simulink library "EOM_lib"  (R2015a)
settings: Solver=ode45  StartTime=0.0  StopTime=10.0  RelTol=1e-3
undefined symbols (not defined in the file): EOM
libraries: aerolibutil x4, aerolib6dof2 x1
settings Model: Creator=Andrew  LastModifiedBy=Andrew

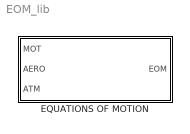
== system EOM_lib ==
  EQUATIONS OF MOTION : Subsystem

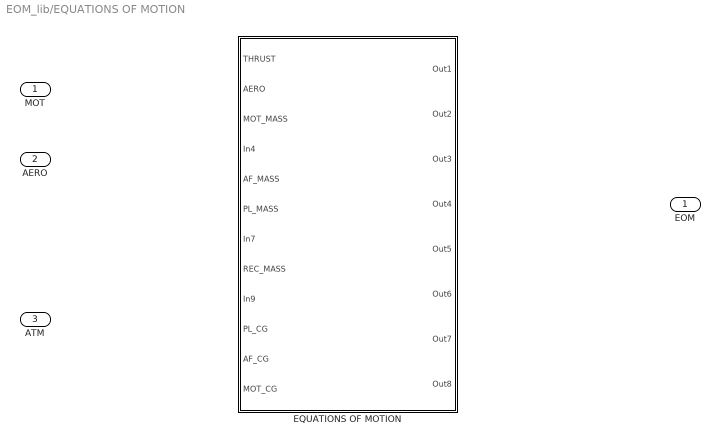
== system EOM_lib/EQUATIONS OF MOTION ==
  MOT : Inport
  AERO : Inport  Port=2
  ATM : Inport  Port=3
  EQUATIONS OF MOTION : Subsystem
  EOM : Outport

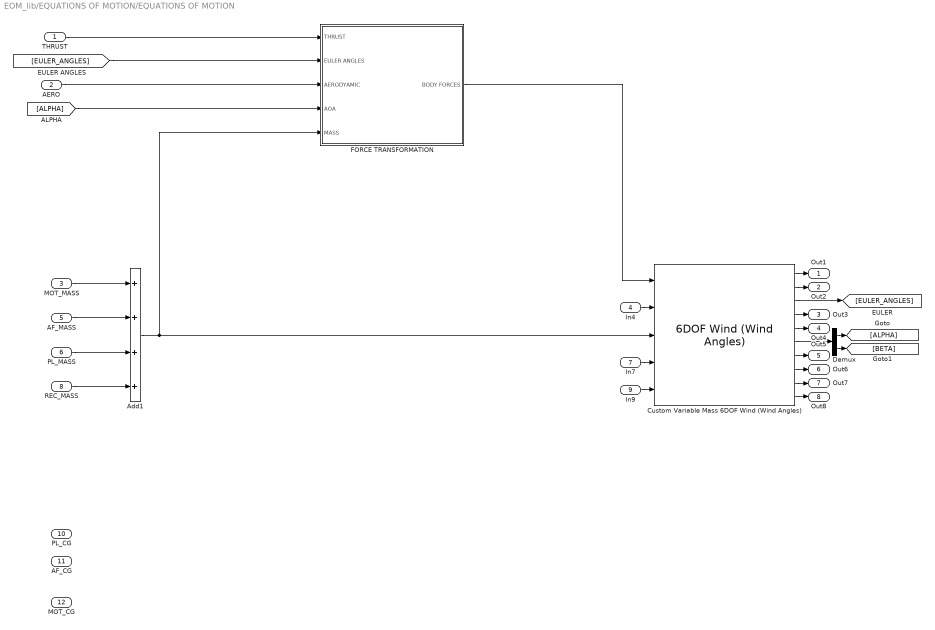
== system EOM_lib/EQUATIONS OF MOTION/EQUATIONS OF MOTION ==
  THRUST : Inport
  AERO : Inport  Port=2
  MOT_MASS : Inport  Port=3
  In4 : Inport  Port=4
  AF_MASS : Inport  Port=5
  PL_MASS : Inport  Port=6
  In7 : Inport  Port=7
  REC_MASS : Inport  Port=8
  In9 : Inport  Port=9
  PL_CG : Inport  Port=10
  AF_CG : Inport  Port=11
  MOT_CG : Inport  Port=12
  Add1 : Sum  Inputs=++++
  Custom Variable Mass 6DOF Wind (Wind Angles) : aerolib6dof2/6DOF Wind (Wind Angles)  units=Metric (MKS)  mtype=Custom Variable  rep=Wind Angles  xme_0=[0 0 0]  Vm_0=[0 0 0]  wind_0=[0 0 0]  pm_0=[0 0 0]  mass_0=1.0  mass_e=0.5  mass_f=2.0  inertia=eye(3)  inertia_e=eye(3)  inertia_f=2*eye(3)  vre_flag=off
  Demux : Demux  Outputs=2
  FORCE TRANSFORMATION : Subsystem
  Out1 : Outport
  Out2 : Outport  Port=2
  Out3 : Outport  Port=3
  Out4 : Outport  Port=4
  Out5 : Outport  Port=5
  Out6 : Outport  Port=6
  Out7 : Outport  Port=7
  Out8 : Outport  Port=8
  wires:
  In4/1 -> Custom Variable Mass 6DOF Wind (Wind Angles)/2
  Demux/1 -> [ALPHA]
  Custom Variable Mass 6DOF Wind (Wind Angles)/3 -> [EULER_ANGLES]
  AF_MASS/1 -> Add1/2
  MOT_MASS/1 -> Add1/1
  PL_MASS/1 -> Add1/3
  Custom Variable Mass 6DOF Wind (Wind Angles)/6 -> Demux/1
  [ALPHA] -> FORCE TRANSFORMATION/4(AOA)
  REC_MASS/1 -> Add1/4
  FORCE TRANSFORMATION/1(BODY FORCES) -> Custom Variable Mass 6DOF Wind (Wind Angles)/1
  [EULER_ANGLES] -> FORCE TRANSFORMATION/2(EULER ANGLES)
  THRUST/1 -> FORCE TRANSFORMATION/1(THRUST)
  Add1/1 -> Custom Variable Mass 6DOF Wind (Wind Angles)/3, FORCE TRANSFORMATION/5(MASS)
  Demux/2 -> [BETA]
  AERO/1 -> FORCE TRANSFORMATION/3(AERODYAMIC)
  Custom Variable Mass 6DOF Wind (Wind Angles)/4 -> Out3/1
  Custom Variable Mass 6DOF Wind (Wind Angles)/10 -> Out8/1
  In9/1 -> Custom Variable Mass 6DOF Wind (Wind Angles)/5
  Custom Variable Mass 6DOF Wind (Wind Angles)/1 -> Out1/1
  Custom Variable Mass 6DOF Wind (Wind Angles)/7 -> Out5/1
  Custom Variable Mass 6DOF Wind (Wind Angles)/2 -> Out2/1
  Custom Variable Mass 6DOF Wind (Wind Angles)/8 -> Out6/1
  In7/1 -> Custom Variable Mass 6DOF Wind (Wind Angles)/4
  Custom Variable Mass 6DOF Wind (Wind Angles)/5 -> Out4/1
  Custom Variable Mass 6DOF Wind (Wind Angles)/9 -> Out7/1

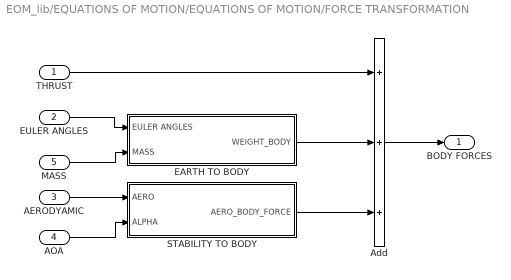
== system EOM_lib/EQUATIONS OF MOTION/EQUATIONS OF MOTION/FORCE TRANSFORMATION ==
  THRUST : Inport
  EULER ANGLES : Inport  Port=2
  AERODYAMIC : Inport  Port=3
  AOA : Inport  Port=4
  MASS : Inport  Port=5
  Add : Sum  Inputs=+++
  EARTH TO BODY : Subsystem
  STABILITY TO BODY : Subsystem
  BODY FORCES : Outport
  wires:
  EULER ANGLES/1 -> EARTH TO BODY/1(EULER ANGLES)
  MASS/1 -> EARTH TO BODY/2(MASS)
  EARTH TO BODY/1(WEIGHT_BODY) -> Add/2
  AERODYAMIC/1 -> STABILITY TO BODY/1(AERO)
  STABILITY TO BODY/1(AERO_BODY_FORCE) -> Add/3
  THRUST/1 -> Add/1
  Add/1 -> BODY FORCES/1
  AOA/1 -> STABILITY TO BODY/2(ALPHA)

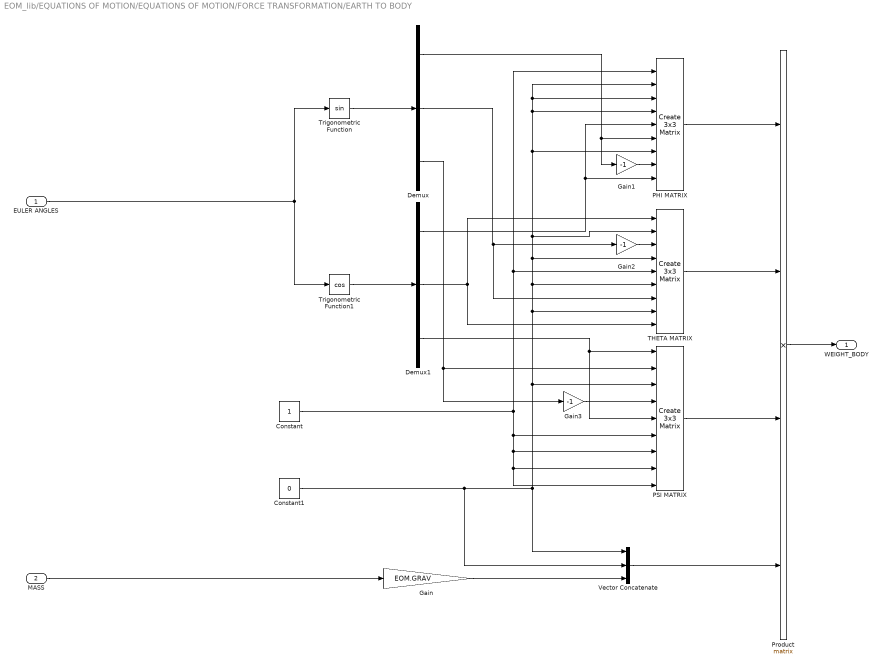
== system EOM_lib/EQUATIONS OF MOTION/EQUATIONS OF MOTION/FORCE TRANSFORMATION/EARTH TO BODY ==
  EULER ANGLES : Inport
  MASS : Inport  Port=2
  Constant : Constant
  Constant1 : Constant  Value=0
  Demux : Demux  Outputs=3
  Demux1 : Demux  Outputs=3
  Gain : Gain  Gain=EOM.GRAV
  Gain1 : Gain  Gain=-1
  Gain2 : Gain  Gain=-1
  Gain3 : Gain  Gain=-1
  "PHI MATRIX " : aerolibutil/Create 3x3 Matrix
  PSI MATRIX : aerolibutil/Create 3x3 Matrix
  Product : Product  Inputs=4  Multiplication=Matrix(*)
  THETA MATRIX : aerolibutil/Create 3x3 Matrix
  Trigonometric Function : Trigonometry
  Trigonometric Function1 : Trigonometry  Operator=cos
  Vector Concatenate : Concatenate  NumInputs=3
  WEIGHT_BODY : Outport
  wires:
  Product/1 -> WEIGHT_BODY/1
  Gain3/1 -> PSI MATRIX/4
  Demux/3 -> PSI MATRIX/2, Gain3/1
  Demux1/3 -> PSI MATRIX/5, PSI MATRIX/1
  Vector Concatenate/1 -> Product/4
  PSI MATRIX/1 -> Product/3
  THETA MATRIX/1 -> Product/2
  "PHI MATRIX "/1 -> Product/1
  MASS/1 -> Gain/1
  Demux/1 -> Gain1/1, "PHI MATRIX "/6
  Gain/1 -> Vector Concatenate/3
  Constant1/1 -> Vector Concatenate/2, Vector Concatenate/1, PSI MATRIX/3, THETA MATRIX/8, THETA MATRIX/6, THETA MATRIX/4, THETA MATRIX/2, "PHI MATRIX "/7, "PHI MATRIX "/4, "PHI MATRIX "/3, "PHI MATRIX "/2
  Trigonometric Function1/1 -> Demux1/1
  Demux1/1 -> "PHI MATRIX "/5, "PHI MATRIX "/9
  Trigonometric Function/1 -> Demux/1
  Demux/2 -> THETA MATRIX/7, Gain2/1
  Demux1/2 -> THETA MATRIX/1, THETA MATRIX/9
  EULER ANGLES/1 -> Trigonometric Function/1, Trigonometric Function1/1
  Gain2/1 -> THETA MATRIX/3
  Gain1/1 -> "PHI MATRIX "/8
  Constant/1 -> PSI MATRIX/7, PSI MATRIX/8, PSI MATRIX/9, PSI MATRIX/6, "PHI MATRIX "/1, THETA MATRIX/5

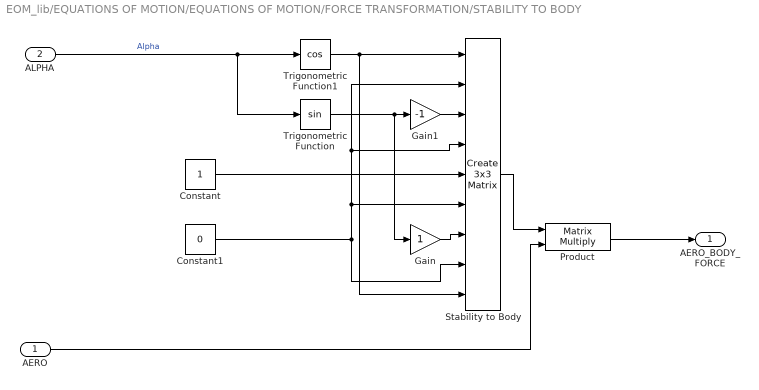
== system EOM_lib/EQUATIONS OF MOTION/EQUATIONS OF MOTION/FORCE TRANSFORMATION/STABILITY TO BODY ==
  AERO : Inport
  ALPHA : Inport  Port=2
  Constant : Constant
  Constant1 : Constant  Value=0
  Gain : Gain
  Gain1 : Gain  Gain=-1
  Product : Product  Multiplication=Matrix(*)
  Stability to Body : aerolibutil/Create 3x3 Matrix
  Trigonometric Function : Trigonometry
  Trigonometric Function1 : Trigonometry  Operator=cos
  AERO_BODY_FORCE : Outport
  wires:
  Gain/1 -> Stability to Body/7
  Trigonometric Function1/1 -> Stability to Body/9, Stability to Body/1
  AERO/1 -> Product/2
  Product/1 -> AERO_BODY_FORCE/1
  Constant1/1 -> Stability to Body/8, Stability to Body/6, Stability to Body/4, Stability to Body/2
  Gain1/1 -> Stability to Body/3
  Trigonometric Function/1 -> Gain/1, Gain1/1
  Constant/1 -> Stability to Body/5
  Stability to Body/1 -> Product/1
  ALPHA/1 -> Trigonometric Function/1, Trigonometric Function1/1  "Alpha"
